simulink model "MaskingPink"  (R2023b)
settings: Solver=FixedStepAuto  StartTime=0.0  StopTime=inf  RelTol=1e-3
libraries: androiduilib x3, androidaudiovideolib x2, dspsrcs4 x1
settings Model: Creator=The MathWorks, Inc.  LastModifiedBy=hp
settings SolverCC: MaxZcPerStep=1
settings OptimizationCC: EnhancedBackFolding=on  PassReuseOutputArgsThreshold=0  MaxStackSize=64  OptimizeBlockOrder=speed  DifferentSizesBufferReuse=on  OptimizationCustomize=off
settings DebuggingCC: ParameterTunabilityLossMsg=error  UnconnectedInputMsg=warning  UnconnectedOutputMsg=warning  UnconnectedLineMsg=warning
settings HardwareCC: ProdBitPerPointer=32  ProdBitPerSizeT=32  ProdBitPerPtrDiffT=32  ProdLargestAtomicInteger=Long  ProdLargestAtomicFloat=Double  ProdWordSize=32  ProdHWDeviceType=ARM Compatible->ARM Cortex  UseEmbeddedCoderFeatures=off  UseSimulinkCoderFeatures=off
settings ModelReferenceCC: EnableRefExpFcnMdlSchedulingChecks=on
settings RTWCC: Description=Embedded Coder  SystemTargetFile=ert.tlc  HardwareBoard=Android Device  TLCOptions="-aInlineSetEventsForThisBaseRateFcn=TLC_FALSE -aSuppressMultiTaskScheduler=TLC_FALSE  -aRateBasedStepFcn=0"  TemplateMakefile=ert_default_tmf  RTWVerbose=off  Toolchain=Android SDK/NDK Tools  DLArmComputeVersion=19.05
settings CodeAppCC: ForceParamTrailComments=on  OperatorAnnotations=on
settings ERTTargetCC: ERTCustomFileBanners=off  SupportContinuousTime=on  SupportNonInlinedSFcns=on  RemoveResetFunc=off  ModelStepFunctionPrototypeControlCompliant=off

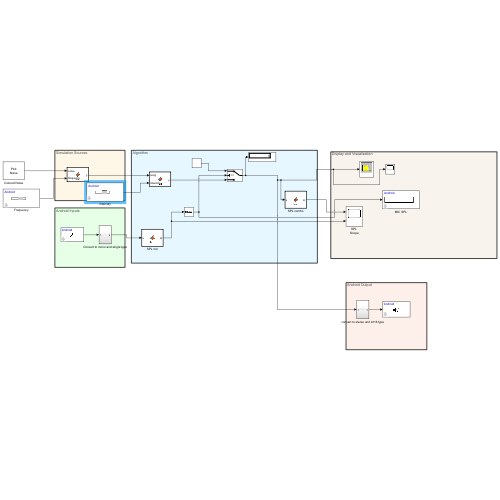
[thumbnail: Simulink's stored preview of the top-level diagram]
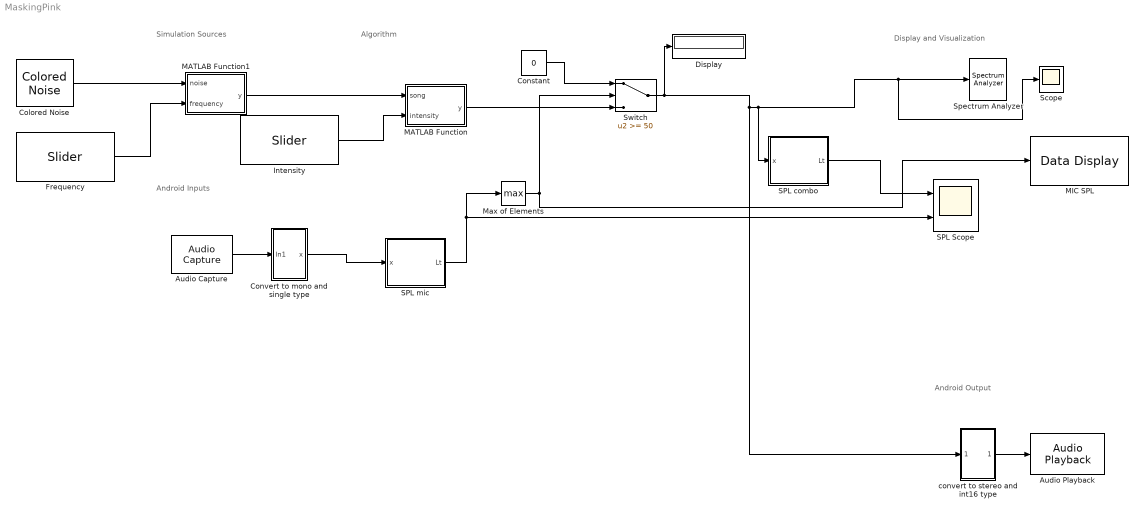
== system MaskingPink ==
  note: Algorithm
  note: Android Inputs
  note: Android Output
  note: Display and Visualization
  note: Simulation Sources
  Audio Capture : androidaudiovideolib/Audio Capture  SampleFreq=44100  FrameSize=4410  SampleTime=0.1  SimulateUsing=Code generation  DeviceStr=0  QueueDuration=0  BlockPlatform=Android  AudioSamplingFreq=44100
  Audio Playback : androidaudiovideolib/Audio Playback  SampleFreq=44100  AudioSamplingFreq=44100  SampleTime=0.1  DeviceStr=0  QueueDuration=0  BlockPlatform=Android
  Colored Noise : dspsrcs4/Colored Noise  Color=pink  InverseFrequencyPower=1  BoundedOutput=on  NumChannels=1  OutputDataType=double  SamplesPerFrame=4410  SampleTime=1  RandomStream=mt19937ar with seed  Seed=67  SimulateUsing=Interpreted execution
      settings: LibrarySourceBlock=audiosources/Colored Noise
  Constant : Constant  Value=0
  Convert to mono and single type : Subsystem
  Display : Display
  Frequency : androiduilib/Slider  Min=20  Value=20  Max=20000  Resolution=1  SliderId=MaskingPink/Frequency  SampleTime=1  BlockPlatform=Android
  Intensity : androiduilib/Slider  Min=0  Value=0  Max=100  Resolution=0.1  SliderId=MaskingPink/Intensity  SampleTime=0.1  BlockPlatform=Android
  MATLAB Function : MATLAB Function  TreatAsAtomicUnit=on
  MATLAB Function1 : MATLAB Function  TreatAsAtomicUnit=on
  MIC SPL : androiduilib/Data Display  DataDisplayId=MaskingPink/MIC_SPL  Format=Float  Precision=6  SimulateUsing=Code generation  blockPlatform=Android
  Max of Elements : MinMax  Function=max
  SPL Scope : Scope  NumInputPorts=2
  SPL combo : MATLAB Function  TreatAsAtomicUnit=on
  SPL mic : MATLAB Function  TreatAsAtomicUnit=on
  Scope : Scope
  Spectrum Analyzer : SpectrumAnalyzer  WindowPosition=[302.000000,321.000000,800.000000,450.000000,]  ScopeFrameLocation=window  SampleRate=44100  Span=44100  StartFrequency=-22050  StopFrequency=22050  AveragingMethod=Exponential  YLimits=[-3603.44492261,-2802.67938425]
  Switch : Switch  Threshold=50  SaturateOnIntegerOverflow=off  InputSameDT=off
  convert to stereo and int16 type : Subsystem
  wires:
  Audio Capture/1 -> Convert to mono and single type/1(In1)
  convert to stereo and int16 type/1(Out1) -> Audio Playback/1
  SPL mic/1(Lt) -> SPL Scope/2, Max of Elements/1
  Convert to mono and single type/1(x) -> SPL mic/1(x)
  Max of Elements/1 -> Switch/2, MIC SPL/1
  Constant/1 -> Switch/1
  SPL combo/1(Lt) -> SPL Scope/1
  Switch/1 -> convert to stereo and int16 type/1(In1), SPL combo/1(x), Scope/1, Spectrum Analyzer/1, Display/1
  Colored Noise/1 -> MATLAB Function1/1(noise)
  MATLAB Function/1(y) -> Switch/3
  MATLAB Function1/1(y) -> MATLAB Function/1(song)
  Frequency/1 -> MATLAB Function1/2(frequency)
  Intensity/1 -> MATLAB Function/2(intensity)

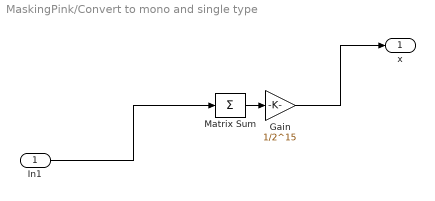
== system MaskingPink/Convert to mono and single type ==
  In1 : Inport
  Gain : Gain  Gain=1/2^15  OutDataTypeStr=single
  Matrix Sum : Sum  Inputs=+  CollapseMode=Specified dimension  CollapseDim=2
  x : Outport
  wires:
  Matrix Sum/1 -> Gain/1
  Gain/1 -> x/1
  In1/1 -> Matrix Sum/1

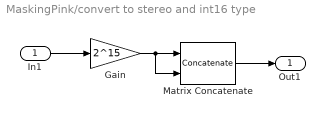
== system MaskingPink/convert to stereo and int16 type ==
  In1 : Inport
  Gain : Gain  Gain=2^15  OutDataTypeStr=int16  SaturateOnIntegerOverflow=on
  Matrix Concatenate : Concatenate  Mode=Multidimensional array  ConcatenateDimension=2
  Out1 : Outport
  wires:
  In1/1 -> Gain/1
  Matrix Concatenate/1 -> Out1/1
  Gain/1 -> Matrix Concatenate/2, Matrix Concatenate/1

== matlab function MaskingPink/SPL mic ==
  data: x input; Lt output
function Lt  = fcn(x)

SPL = splMeter(TimeWeighting="Fast", ...
    FrequencyWeighting="A-weighting", ...
    SampleRate=44100, ...
    TimeInterval=2);
% Lt = zeros(size(x)); 
% [Lt,Leq,Lpeak,Lmax] = SPL(x);

Lt= SPL(x);

== matlab function MaskingPink/SPL combo ==
  data: x input; Lt output
function Lt  = fcn(x)

SPL = splMeter(TimeWeighting="Fast", ...
    FrequencyWeighting="A-weighting", ...
    SampleRate=44100, ...
    TimeInterval=10);
% Lt = zeros(size(x)); 
% [Lt,Leq,Lpeak,Lmax] = SPL(x);

Lt= SPL(x);

== matlab function MaskingPink/MATLAB Function ==
  data: song input; y output; intensity input
function y = fcn(song,intensity)

y = song*(intensity+5)/100;

== matlab function MaskingPink/MATLAB Function1 ==
  data: noise input; y output; frequency input
function y = fcn(noise,frequency)
% Define parameters
numSamples = 4410; % Number of samples


% Low-pass filter parameters
windowSize = 44100/(2*(2*frequency/3)); % Window size for moving average

% Apply the moving average filter without using functions
filteredSignal = zeros(numSamples,1);

for i = 1:numSamples
    if i <= windowSize
        % For the initial samples, the filter covers only available data
        filteredSignal(i) = mean(noise(1:i));
    else
        % For the rest of the samples, apply the moving average window
        filteredSignal(i) = mean(noise(i-windowSize+1:i));
    end
end
y = filteredSignal;
